simulink model "RippleCntSwArch"  (R2021b)
settings: Solver=FixedStepDiscrete  StartTime=0.0  StopTime=10.0  RelTol=1e-3
settings Model: Creator=JYOUNG16  LastModifiedBy=JYOUNG16

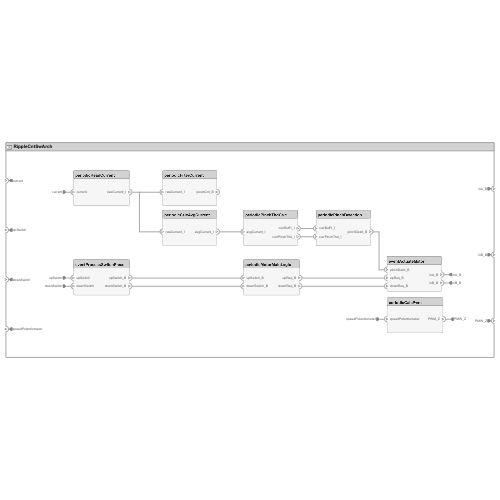
[thumbnail: Simulink's stored preview of the top-level diagram]
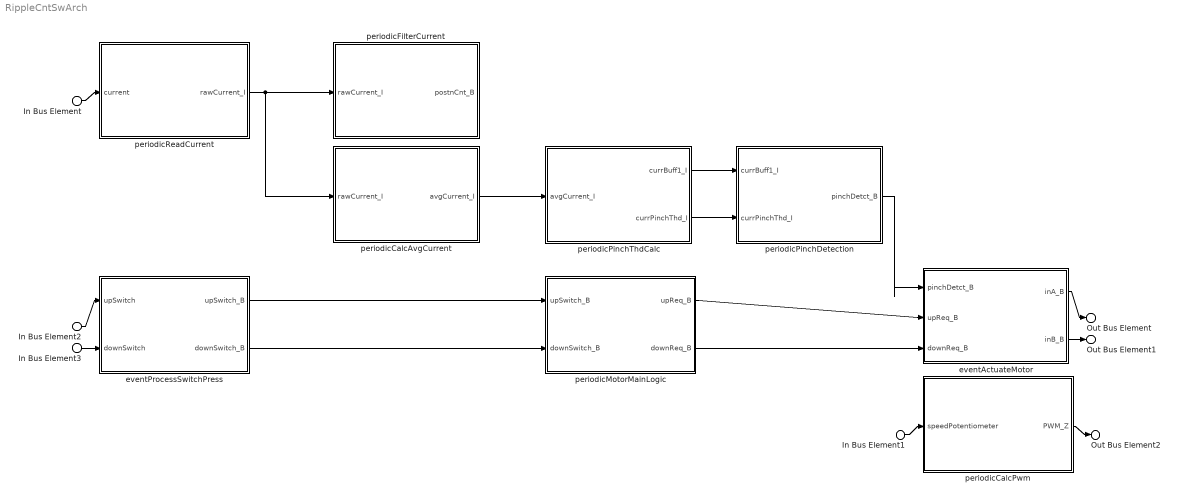
== system RippleCntSwArch ==
  In Bus Element : Inport  PortName=current
  In Bus Element2 : Inport  Port=2  PortName=upSwitch
  In Bus Element3 : Inport  Port=3  PortName=downSwitch
  In Bus Element1 : Inport  Port=4  PortName=speedPotentiometer
  eventActuateMotor : Subsystem
      settings: PortSchema="{\"entries\":[{\"content\":{\"headerSize\":26,\"margin\":15,\"minimumSpacing\":25,\"sides\":[{\"content\":{\"connectorIds\":[\"In1\",\"In2\",\"In3\"]},\"type\":\"ConnectorPlacement.EquallySpacedRectSide\",\"uuid\":\"e90e293d-51f3-41d3-acba-cceb8fcb60e2\"},{\"content\":{\"connectorIds\":[\"Out1\",\"Out2\"],\"side\":\"RIGHT\"},\"type\":\"ConnectorPlacement.EquallySpacedRectSide\",\"uuid\":\"67eac8de-18f9-484b-9c44-0eefaf548d79\"},{\"content\":{\"connectorIds\":[],\"side\":\"TOP\"},\"type\":\"ConnectorPlacement.EquallySpacedRectSide\",\"uuid\":\"4158b683-0d0e-4b89-b83e-901791eae0e7\"}]},\"type\":\"ConnectorPlacement.EquallySpacedConnector\",\"uuid\":\"58e86cb2-f041-4342-8ce6-994764ef79de\"}],\"packageUris\":[\"http://schema.mathworks.com/mf0/Connector/R2020b\"],\"version\":\"1.0\"}"
  eventProcessSwitchPress : Subsystem
      settings: PortSchema="{\"entries\":[{\"content\":{\"headerSize\":26,\"margin\":15,\"minimumSpacing\":25,\"sides\":[{\"content\":{\"connectorIds\":[\"In1\",\"In2\"]},\"type\":\"ConnectorPlacement.EquallySpacedRectSide\",\"uuid\":\"e90e293d-51f3-41d3-acba-cceb8fcb60e2\"},{\"content\":{\"connectorIds\":[\"Out1\",\"Out2\"],\"side\":\"RIGHT\"},\"type\":\"ConnectorPlacement.EquallySpacedRectSide\",\"uuid\":\"67eac8de-18f9-484b-9c44-0eefaf548d79\"},{\"content\":{\"connectorIds\":[],\"side\":\"TOP\"},\"type\":\"ConnectorPlacement.EquallySpacedRectSide\",\"uuid\":\"4158b683-0d0e-4b89-b83e-901791eae0e7\"}]},\"type\":\"ConnectorPlacement.EquallySpacedConnector\",\"uuid\":\"58e86cb2-f041-4342-8ce6-994764ef79de\"}],\"packageUris\":[\"http://schema.mathworks.com/mf0/Connector/R2020b\"],\"version\":\"1.0\"}"
  periodicCalcAvgCurrent : Subsystem
      settings: PortSchema="{\"entries\":[{\"content\":{\"headerSize\":26,\"margin\":15,\"minimumSpacing\":25,\"sides\":[{\"content\":{\"connectorIds\":[\"In1\"]},\"type\":\"ConnectorPlacement.EquallySpacedRectSide\",\"uuid\":\"e90e293d-51f3-41d3-acba-cceb8fcb60e2\"},{\"content\":{\"connectorIds\":[\"Out1\"],\"side\":\"RIGHT\"},\"type\":\"ConnectorPlacement.EquallySpacedRectSide\",\"uuid\":\"67eac8de-18f9-484b-9c44-0eefaf548d79\"},{\"content\":{\"connectorIds\":[],\"side\":\"TOP\"},\"type\":\"ConnectorPlacement.EquallySpacedRectSide\",\"uuid\":\"4158b683-0d0e-4b89-b83e-901791eae0e7\"}]},\"type\":\"ConnectorPlacement.EquallySpacedConnector\",\"uuid\":\"58e86cb2-f041-4342-8ce6-994764ef79de\"}],\"packageUris\":[\"http://schema.mathworks.com/mf0/Connector/R2020b\"],\"version\":\"1.0\"}"
  periodicCalcPwm : Subsystem
      settings: PortSchema="{\"entries\":[{\"content\":{\"headerSize\":26,\"margin\":15,\"minimumSpacing\":25,\"sides\":[{\"content\":{\"connectorIds\":[\"In1\"]},\"type\":\"ConnectorPlacement.EquallySpacedRectSide\",\"uuid\":\"e90e293d-51f3-41d3-acba-cceb8fcb60e2\"},{\"content\":{\"connectorIds\":[\"Out1\"],\"side\":\"RIGHT\"},\"type\":\"ConnectorPlacement.EquallySpacedRectSide\",\"uuid\":\"67eac8de-18f9-484b-9c44-0eefaf548d79\"},{\"content\":{\"connectorIds\":[],\"side\":\"TOP\"},\"type\":\"ConnectorPlacement.EquallySpacedRectSide\",\"uuid\":\"4158b683-0d0e-4b89-b83e-901791eae0e7\"}]},\"type\":\"ConnectorPlacement.EquallySpacedConnector\",\"uuid\":\"58e86cb2-f041-4342-8ce6-994764ef79de\"}],\"packageUris\":[\"http://schema.mathworks.com/mf0/Connector/R2020b\"],\"version\":\"1.0\"}"
  periodicFilterCurrent : Subsystem
      settings: PortSchema="{\"entries\":[{\"content\":{\"headerSize\":26,\"margin\":15,\"minimumSpacing\":25,\"sides\":[{\"content\":{\"connectorIds\":[\"In1\"]},\"type\":\"ConnectorPlacement.EquallySpacedRectSide\",\"uuid\":\"e90e293d-51f3-41d3-acba-cceb8fcb60e2\"},{\"content\":{\"connectorIds\":[\"Out1\"],\"side\":\"RIGHT\"},\"type\":\"ConnectorPlacement.EquallySpacedRectSide\",\"uuid\":\"67eac8de-18f9-484b-9c44-0eefaf548d79\"},{\"content\":{\"connectorIds\":[],\"side\":\"TOP\"},\"type\":\"ConnectorPlacement.EquallySpacedRectSide\",\"uuid\":\"4158b683-0d0e-4b89-b83e-901791eae0e7\"}]},\"type\":\"ConnectorPlacement.EquallySpacedConnector\",\"uuid\":\"58e86cb2-f041-4342-8ce6-994764ef79de\"}],\"packageUris\":[\"http://schema.mathworks.com/mf0/Connector/R2020b\"],\"version\":\"1.0\"}"
  periodicMotorMainLogic : Subsystem
      settings: PortSchema="{\"entries\":[{\"content\":{\"headerSize\":26,\"margin\":15,\"minimumSpacing\":25,\"sides\":[{\"content\":{\"connectorIds\":[\"In1\",\"In2\"]},\"type\":\"ConnectorPlacement.EquallySpacedRectSide\",\"uuid\":\"e90e293d-51f3-41d3-acba-cceb8fcb60e2\"},{\"content\":{\"connectorIds\":[\"Out1\",\"Out2\"],\"side\":\"RIGHT\"},\"type\":\"ConnectorPlacement.EquallySpacedRectSide\",\"uuid\":\"67eac8de-18f9-484b-9c44-0eefaf548d79\"},{\"content\":{\"connectorIds\":[],\"side\":\"TOP\"},\"type\":\"ConnectorPlacement.EquallySpacedRectSide\",\"uuid\":\"4158b683-0d0e-4b89-b83e-901791eae0e7\"}]},\"type\":\"ConnectorPlacement.EquallySpacedConnector\",\"uuid\":\"58e86cb2-f041-4342-8ce6-994764ef79de\"}],\"packageUris\":[\"http://schema.mathworks.com/mf0/Connector/R2020b\"],\"version\":\"1.0\"}"
  periodicPinchDetection : Subsystem
      settings: PortSchema="{\"entries\":[{\"content\":{\"headerSize\":26,\"margin\":15,\"minimumSpacing\":25,\"sides\":[{\"content\":{\"connectorIds\":[\"In1\",\"In2\"]},\"type\":\"ConnectorPlacement.EquallySpacedRectSide\",\"uuid\":\"e90e293d-51f3-41d3-acba-cceb8fcb60e2\"},{\"content\":{\"connectorIds\":[\"Out1\"],\"side\":\"RIGHT\"},\"type\":\"ConnectorPlacement.EquallySpacedRectSide\",\"uuid\":\"67eac8de-18f9-484b-9c44-0eefaf548d79\"},{\"content\":{\"connectorIds\":[],\"side\":\"TOP\"},\"type\":\"ConnectorPlacement.EquallySpacedRectSide\",\"uuid\":\"4158b683-0d0e-4b89-b83e-901791eae0e7\"}]},\"type\":\"ConnectorPlacement.EquallySpacedConnector\",\"uuid\":\"58e86cb2-f041-4342-8ce6-994764ef79de\"}],\"packageUris\":[\"http://schema.mathworks.com/mf0/Connector/R2020b\"],\"version\":\"1.0\"}"
  periodicPinchThdCalc : Subsystem
      settings: PortSchema="{\"entries\":[{\"content\":{\"headerSize\":26,\"margin\":15,\"minimumSpacing\":25,\"sides\":[{\"content\":{\"connectorIds\":[\"In1\"]},\"type\":\"ConnectorPlacement.EquallySpacedRectSide\",\"uuid\":\"e90e293d-51f3-41d3-acba-cceb8fcb60e2\"},{\"content\":{\"connectorIds\":[\"Out1\",\"Out2\"],\"side\":\"RIGHT\"},\"type\":\"ConnectorPlacement.EquallySpacedRectSide\",\"uuid\":\"67eac8de-18f9-484b-9c44-0eefaf548d79\"},{\"content\":{\"connectorIds\":[],\"side\":\"TOP\"},\"type\":\"ConnectorPlacement.EquallySpacedRectSide\",\"uuid\":\"4158b683-0d0e-4b89-b83e-901791eae0e7\"}]},\"type\":\"ConnectorPlacement.EquallySpacedConnector\",\"uuid\":\"58e86cb2-f041-4342-8ce6-994764ef79de\"}],\"packageUris\":[\"http://schema.mathworks.com/mf0/Connector/R2020b\"],\"version\":\"1.0\"}"
  periodicReadCurrent : Subsystem
      settings: PortSchema="{\"entries\":[{\"content\":{\"headerSize\":26,\"margin\":15,\"minimumSpacing\":25,\"sides\":[{\"content\":{\"connectorIds\":[\"In1\"]},\"type\":\"ConnectorPlacement.EquallySpacedRectSide\",\"uuid\":\"e90e293d-51f3-41d3-acba-cceb8fcb60e2\"},{\"content\":{\"connectorIds\":[\"Out1\"],\"side\":\"RIGHT\"},\"type\":\"ConnectorPlacement.EquallySpacedRectSide\",\"uuid\":\"67eac8de-18f9-484b-9c44-0eefaf548d79\"},{\"content\":{\"connectorIds\":[],\"side\":\"TOP\"},\"type\":\"ConnectorPlacement.EquallySpacedRectSide\",\"uuid\":\"4158b683-0d0e-4b89-b83e-901791eae0e7\"}]},\"type\":\"ConnectorPlacement.EquallySpacedConnector\",\"uuid\":\"58e86cb2-f041-4342-8ce6-994764ef79de\"}],\"packageUris\":[\"http://schema.mathworks.com/mf0/Connector/R2020b\"],\"version\":\"1.0\"}"
  Out Bus Element : Outport  PortName=inA_B
  Out Bus Element1 : Outport  Port=2  PortName=inB_B
  Out Bus Element2 : Outport  Port=3  PortName=PMW_Z
  wires:
  periodicReadCurrent/1(rawCurrent_I) -> periodicCalcAvgCurrent/1(rawCurrent_I), periodicFilterCurrent/1(rawCurrent_I)
  periodicMotorMainLogic/1(upReq_B) -> eventActuateMotor/2(upReq_B)
  periodicMotorMainLogic/2(downReq_B) -> eventActuateMotor/3(downReq_B)
  periodicCalcAvgCurrent/1(avgCurrent_I) -> periodicPinchThdCalc/1(avgCurrent_I)
  eventActuateMotor/1(inA_B) -> Out Bus Element/1
  eventActuateMotor/2(inB_B) -> Out Bus Element1/1
  periodicCalcPwm/1(PWM_Z) -> Out Bus Element2/1
  periodicPinchThdCalc/1(currBuff1_I) -> periodicPinchDetection/1(currBuff1_I)
  periodicPinchThdCalc/2(currPinchThd_I) -> periodicPinchDetection/2(currPinchThd_I)
  periodicPinchDetection/1(pinchDetct_B) -> eventActuateMotor/1(pinchDetct_B)
  In Bus Element/1 -> periodicReadCurrent/1(current)
  In Bus Element2/1 -> eventProcessSwitchPress/1(upSwitch)
  In Bus Element3/1 -> eventProcessSwitchPress/2(downSwitch)
  In Bus Element1/1 -> periodicCalcPwm/1(speedPotentiometer)
  eventProcessSwitchPress/1(upSwitch_B) -> periodicMotorMainLogic/1(upSwitch_B)
  eventProcessSwitchPress/2(downSwitch_B) -> periodicMotorMainLogic/2(downSwitch_B)

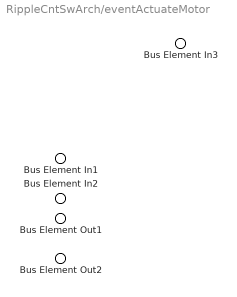
== system RippleCntSwArch/eventActuateMotor ==
  Bus Element In3 : Inport  PortName=pinchDetct_B
  Bus Element In1 : Inport  Port=2  PortName=upReq_B
  Bus Element In2 : Inport  Port=3  PortName=downReq_B
  Bus Element Out1 : Outport  PortName=inA_B
  Bus Element Out2 : Outport  Port=2  PortName=inB_B

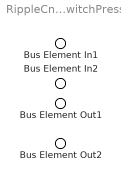
== system RippleCntSwArch/eventProcessSwitchPress ==
  Bus Element In1 : Inport  PortName=upSwitch
  Bus Element In2 : Inport  Port=2  PortName=downSwitch
  Bus Element Out1 : Outport  PortName=upSwitch_B
  Bus Element Out2 : Outport  Port=2  PortName=downSwitch_B

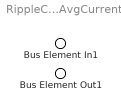
== system RippleCntSwArch/periodicCalcAvgCurrent ==
  Bus Element In1 : Inport  PortName=rawCurrent_I
  Bus Element Out1 : Outport  PortName=avgCurrent_I

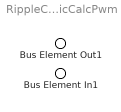
== system RippleCntSwArch/periodicCalcPwm ==
  Bus Element In1 : Inport  PortName=speedPotentiometer
  Bus Element Out1 : Outport  PortName=PWM_Z

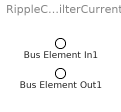
== system RippleCntSwArch/periodicFilterCurrent ==
  Bus Element In1 : Inport  PortName=rawCurrent_I
  Bus Element Out1 : Outport  PortName=postnCnt_B

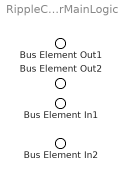
== system RippleCntSwArch/periodicMotorMainLogic ==
  Bus Element In1 : Inport  PortName=upSwitch_B
  Bus Element In2 : Inport  Port=2  PortName=downSwitch_B
  Bus Element Out1 : Outport  PortName=upReq_B
  Bus Element Out2 : Outport  Port=2  PortName=downReq_B

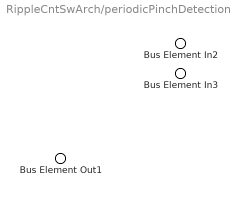
== system RippleCntSwArch/periodicPinchDetection ==
  Bus Element In2 : Inport  PortName=currBuff1_I
  Bus Element In3 : Inport  Port=2  PortName=currPinchThd_I
  Bus Element Out1 : Outport  PortName=pinchDetct_B

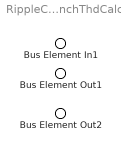
== system RippleCntSwArch/periodicPinchThdCalc ==
  Bus Element In1 : Inport  PortName=avgCurrent_I
  Bus Element Out1 : Outport  PortName=currBuff1_I
  Bus Element Out2 : Outport  Port=2  PortName=currPinchThd_I

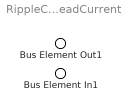
== system RippleCntSwArch/periodicReadCurrent ==
  Bus Element In1 : Inport  PortName=current
  Bus Element Out1 : Outport  PortName=rawCurrent_I
